simulink model "motorDistCtrl_start"  (R2017a)
settings: Solver=VariableStepAuto  StartTime=0.0  StopTime=10.0  RelTol=1e-3
values from neighbouring files (symbols this model uses):
  ticksPerRot = 627.2    [robotParameters.m]
  wheelR = 0.052    [robotParameters.m]
undefined symbols (not defined in the file or in its folder): motorIp, motorSp
libraries: mobileRoboticsTrainingLib x1
settings Model: Creator=sseshadr  LastModifiedBy=shiremat

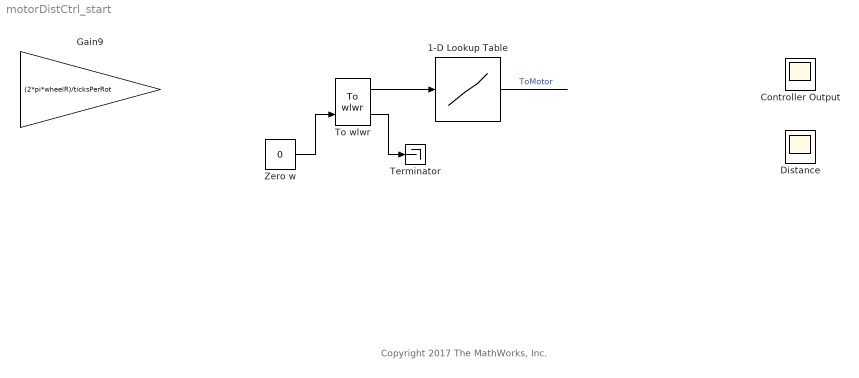
== system motorDistCtrl_start ==
  note: Copyright 2017 The MathWorks, Inc.
  1-D Lookup Table : Lookup_n-D  NumberOfTableDimensions=1  BreakpointsForDimension1=motorSp  Table=motorIp  ExtrapMethod=Clip  InternalRulePriority=Speed  RndMeth=Simplest  InputSameDT=on
  Controller Output : Scope
  Distance : Scope  NumInputPorts=2
  Gain9 : Gain  Gain=(2*pi*wheelR)/ticksPerRot
  Terminator : Terminator
  To wlwr : mobileRoboticsTrainingLib/To wlwr  axleLength=axleLength  wheelR=wheelR
  Zero w : Constant  Value=0
  wires:
  ? -> Distance/1  "Reference"
  ? -> Distance/2  "Measured"
  To wlwr/1 -> 1-D Lookup Table/1
  Zero w/1 -> To wlwr/2
  To wlwr/2 -> Terminator/1
  ? -> Controller Output/1  "Controller"
  ? -> To wlwr/1  "FromPID"
  1-D Lookup Table/1 -> ?  "ToMotor"
